simulink model "Sim2"  (R2016a)
settings: Solver=VariableStepAuto  StartTime=0.0  StopTime=30  RelTol=1e-3
values from neighbouring files (symbols this model uses):
  A = [0 1 0 0 ... (first row only)    [Calculations_veri.m]
  B = [0; 1/J1; 0; 0;]    [Calculations_veri.m]
  C = eye(4)    [Calculations_veri.m]
  D = [0;0;0;0;]    [Calculations_veri.m]
undefined symbols (not defined in the file or in its folder): k
settings Model: Creator=ramik  LastModifiedBy=ra_kand

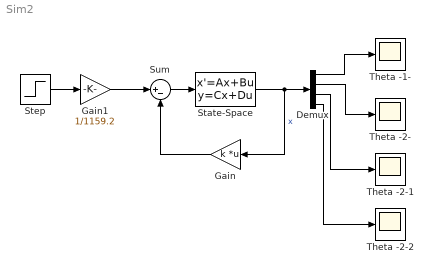
== system Sim2 ==
  Demux : Demux
  Gain : Gain  Gain=k  Multiplication=Matrix(K*u)  OutDataTypeStr=Inherit: Same as input
  Gain1 : Gain  Gain=1/1159.2  OutDataTypeStr=Inherit: Same as input
  State-Space : StateSpace  A=A  B=B  C=C  D=D  X0=0
  Step : Step  SampleTime=0
  Sum : Sum  Inputs=|+-
  Theta -1- : Scope
  Theta -2- : Scope
  Theta -2-1 : Scope
  Theta -2-2 : Scope
  wires:
  Demux/1 -> Theta -1-/1
  Demux/2 -> Theta -2-/1
  State-Space/1 -> Gain/1, Demux/1  "x"
  Demux/3 -> Theta -2-1/1
  Demux/4 -> Theta -2-2/1
  Gain/1 -> Sum/2
  Sum/1 -> State-Space/1
  Step/1 -> Gain1/1
  Gain1/1 -> Sum/1
